simulink model "lazo_abierto"  (R2019a)
settings: Solver=VariableStepAuto  StartTime=0.0  StopTime=50.0  RelTol=1e-3
values from neighbouring files (symbols this model uses):
  den = [34709393649091889, 8873737467196072166715, 24583972753858281030182000, 42460474904292344280000000]    [motor_generador_sim.m]
  K_h = 1.58    [motor_generador_sim.m]
  K_s = 0.003    [motor_generador_sim.m]
  num = [143134928095778949120000, 36192688961361248563200000000]    [motor_generador_sim.m]
  T_h = 0.47    [motor_generador_sim.m]
libraries: simulink x1, simulink_extras x1
settings Model: Creator=lakat  LastModifiedBy=lakat

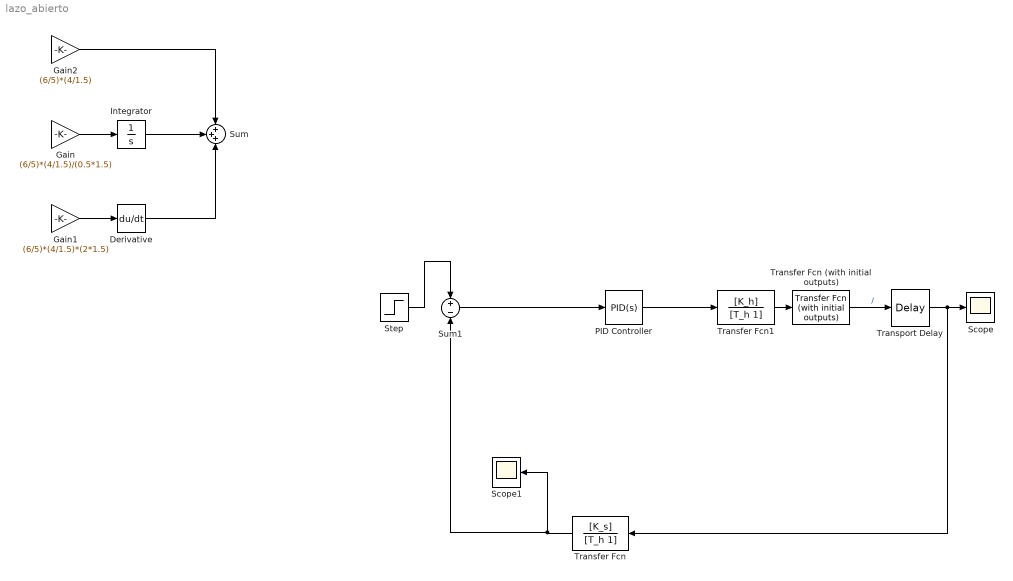
== system lazo_abierto ==
  Derivative : Derivative  CoefficientInTFapproximation=0
  Gain : Gain  Gain=(6/5)*(4/1.5)/(0.5*1.5)
  Gain1 : Gain  Gain=(6/5)*(4/1.5)*(2*1.5)
  Gain2 : Gain  Gain=(6/5)*(4/1.5)
  Integrator : Integrator
  PID Controller : simulink/Continuous/PID Controller  Controller=PID  Form=Parallel  TimeDomain=Continuous-time  SampleTime=-1  IntegratorMethod=Forward Euler  FilterMethod=Forward Euler  ControllerParametersSource=internal  P=(6/5)*(4/1.5)  I=(6/5)*(4/1.5)/(0.5*1.5)  D=0  UseFilter=on  N=0  TunerSelectOption=Transfer Function Based (PID Tuner App)  InitialConditionSource=internal  InitialConditionForIntegrator=0  InitialConditionForFilter=0  DifferentiatorICPrevScaledInput=0  ExternalReset=none  TrackingMode=off  Kt=1  LimitOutput=off  UpperSaturationLimit=inf  LowerSaturationLimit=-inf  LinearizeAsGain=on  AntiWindupMode=none  Kb=1  POutMin=[]  POutMax=[]  IOutMin=[]  IOutMax=[]  DOutMin=[]  DOutMax=[]  NOutMin=[]  NOutMax=[]  SumOutMin=[]  SumOutMax=[]  SaturationOutMin=[]  SaturationOutMax=[]  PParamMin=[]  PParamMax=[]  IParamMin=[]  IParamMax=[]  DParamMin=[]  DParamMax=[]  NParamMin=[]  NParamMax=[]  KbParamMin=[]  KbParamMax=[]  KtParamMin=[]  KtParamMax=[]  KbOutMin=[]  KbOutMax=[]  KtOutMin=[]  KtOutMax=[]  IntegratorOutMin=[]  IntegratorOutMax=[]  FilterOutMin=[]  FilterOutMax=[]  SumI1OutMin=[]  SumI1OutMax=[]  SumI2OutMin=[]  SumI2OutMax=[]  SumI3OutMin=[]  SumI3OutMax=[]  SumI4OutMin=[]  SumI4OutMax=[]  SumDOutMin=[]  SumDOutMax=[]  DifferentiatorOutMin=[]  DifferentiatorOutMax=[]  FilterDiffOutCoefMin=[]  FilterDiffOutCoefMax=[]  ReciprocalOutMin=[]  ReciprocalOutMax=[]  SumDenOutMin=[]  SumDenOutMax=[]  SumNumOutMin=[]  SumNumOutMax=[]  DivideOutMin=[]  DivideOutMax=[]  IntegratorContinuousStateAttributes=''  IntegratorStateMustResolveToSignalObject=off  IntegratorRTWStateStorageClass=Auto  FilterContinuousStateAttributes=''  FilterStateMustResolveToSignalObject=off  FilterRTWStateStorageClass=Auto  ParallelPVariant=InternalParameters  IdealPVariant=Disabled  IVariant=InternalParameters  DVariant=InternalParameters  IntegratorVariant=Continuous  SatVariant=Disabled  AWVariant=Passthrough  PCopyVariant=Disabled  TRVariant=Disabled  FdbkBlocksVariant=Forward  IdealPFdbkVariant=Disabled  SatFdbkVariant=Disabled  DerivativeFilterVariant=ContFilter  NVariant=InternalParameters  NCopyVariant=Disabled  FilterICVariant=InternalICsFilter  IntegratorICVariant=InternalICs  ExternalResetVariant=Disabled  TRSumVariant=Passthrough  SumFdbkVariant=Disabled  SumVariant=Sum_PID
  Scope : Scope
  Scope1 : Scope
  Step : Step  SampleTime=0
  Sum : Sum  Inputs=3
  Sum1 : Sum  Inputs=+-
  Transfer Fcn : TransferFcn  Description=Sensor  Numerator=[K_s]  Denominator=[T_h 1]  ContinuousStateAttributes='sensor'
  Transfer Fcn (with initial outputs) : simulink_extras/Additional Linear/Transfer Fcn (with initial outputs)  Description=Función de transferencia del sistema, con las condiciones iniciales  N=num  D=den  Y0=1500  U0=2
  Transfer Fcn1 : TransferFcn  Numerator=[K_h]  Denominator=[T_h 1]  ContinuousStateAttributes='convertidor'
  Transport Delay : TransportDelay  DelayTime=0.1
  wires:
  Integrator/1 -> Sum/2
  Derivative/1 -> Sum/3
  Gain/1 -> Integrator/1
  Gain1/1 -> Derivative/1
  Gain2/1 -> Sum/1
  Transfer Fcn (with initial outputs)/1 -> Transport Delay/1  "/"
  Transfer Fcn1/1 -> Transfer Fcn (with initial outputs)/1
  Transfer Fcn/1 -> Sum1/2, Scope1/1
  Transport Delay/1 -> Scope/1, Transfer Fcn/1
  Step/1 -> Sum1/1
  PID Controller/1 -> Transfer Fcn1/1
  Sum1/1 -> PID Controller/1
